simulink model "dcMotorControlSimPIDcode_2018b"  (R2018b)
settings: Solver=ode15s  StartTime=0.0  StopTime=10.0  RelTol=1e-3
PreLoadFcn:
  | dcMotorControlInit
undefined symbols (not defined in the file): sampleTime
libraries: fl_lib x16, nesl_utility x8, elec_lib x4, simulink x1, sdl_lib x1
Description:
  | DC Motor Control Simulation
settings Model: Creator=ControlLab  LastModifiedBy=arkadira
settings DataIOCC: SaveFormat=Array  SaveOutput=off  SignalLogging=off  DSMLogging=off  SaveTime=off

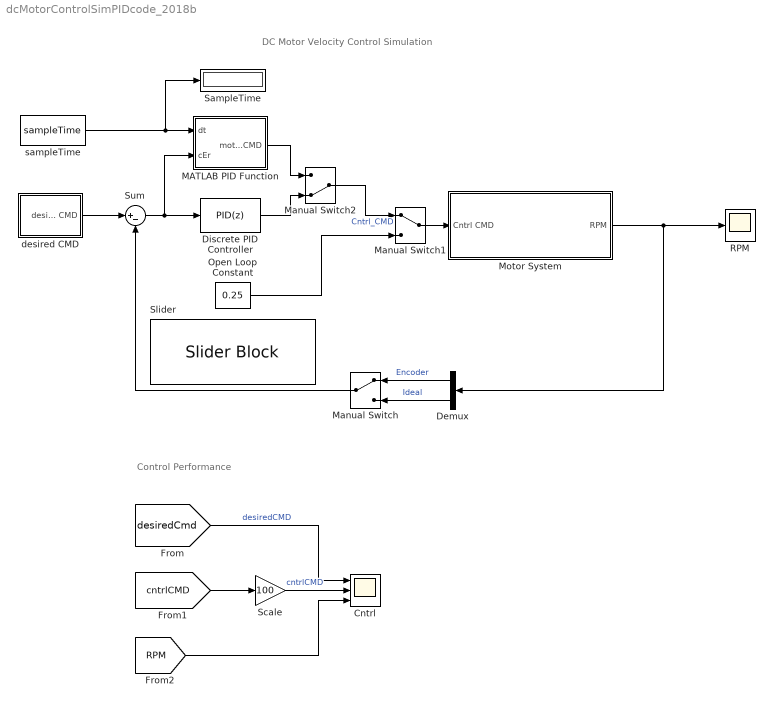
== system dcMotorControlSimPIDcode_2018b ==
  note: Control Performance
  note: DC Motor Velocity Control Simulation
  Cntrl : Scope  NumInputPorts=3
  Demux : Demux  Outputs=2
  Discrete PID Controller : simulink/Continuous/PID Controller  Controller=PID  Form=Parallel  TimeDomain=Discrete-time  SampleTime=sampleTime  IntegratorMethod=Forward Euler  FilterMethod=Forward Euler  ControllerParametersSource=internal  P=0.025  I=0.05  D=0.0001  UseFilter=off  N=0  TunerSelectOption=Transfer Function Based (PID Tuner App)  InitialConditionSource=internal  InitialConditionForIntegrator=0  InitialConditionForFilter=0  DifferentiatorICPrevScaledInput=0  ExternalReset=none  TrackingMode=off  Kt=1  LimitOutput=on  UpperSaturationLimit=1  LowerSaturationLimit=-1  LinearizeAsGain=on  AntiWindupMode=back-calculation  Kb=1  POutMin=[]  POutMax=[]  IOutMin=[]  IOutMax=[]  DOutMin=[]  DOutMax=[]  NOutMin=[]  NOutMax=[]  SumOutMin=[]  SumOutMax=[]  SaturationOutMin=[]  SaturationOutMax=[]  PParamMin=[]  PParamMax=[]  IParamMin=[]  IParamMax=[]  DParamMin=[]  DParamMax=[]  NParamMin=[]  NParamMax=[]  KbParamMin=[]  KbParamMax=[]  KtParamMin=[]  KtParamMax=[]  KbOutMin=[]  KbOutMax=[]  KtOutMin=[]  KtOutMax=[]  IntegratorOutMin=[]  IntegratorOutMax=[]  FilterOutMin=[]  FilterOutMax=[]  SumI1OutMin=[]  SumI1OutMax=[]  SumI2OutMin=[]  SumI2OutMax=[]  SumI3OutMin=[]  SumI3OutMax=[]  SumI4OutMin=[]  SumI4OutMax=[]  SumDOutMin=[]  SumDOutMax=[]  DifferentiatorOutMin=[]  DifferentiatorOutMax=[]  FilterDiffOutCoefMin=[]  FilterDiffOutCoefMax=[]  ReciprocalOutMin=[]  ReciprocalOutMax=[]  SumDenOutMin=[]  SumDenOutMax=[]  SumNumOutMin=[]  SumNumOutMax=[]  DivideOutMin=[]  DivideOutMax=[]  IntegratorContinuousStateAttributes=''  IntegratorStateMustResolveToSignalObject=off  IntegratorRTWStateStorageClass=Auto  FilterContinuousStateAttributes=''  FilterStateMustResolveToSignalObject=off  FilterRTWStateStorageClass=Auto  ParallelPVariant=InternalParameters  IdealPVariant=Disabled  IVariant=InternalParameters  DVariant=InternalParameters  IntegratorVariant=Discrete  SatVariant=Enabled  AWVariant=BackCalculation  PCopyVariant=Disabled  TRVariant=Disabled  FdbkBlocksVariant=Forward  IdealPFdbkVariant=Disabled  SatFdbkVariant=Disabled  DerivativeFilterVariant=Differentiator  NVariant=Passthrough  NCopyVariant=Disabled_SignalSpec  FilterICVariant=InternalICsDifferentiator  IntegratorICVariant=InternalICs  ExternalResetVariant=Disabled  TRSumVariant=Passthrough  SumFdbkVariant=Disabled  SumVariant=Sum_PID
  MATLAB PID Function : MATLAB Function  TreatAsAtomicUnit=on  SystemSampleTime=sampleTime
  Manual Switch : ManualSwitch
  Manual Switch1 : ManualSwitch
  Manual Switch2 : ManualSwitch  CurrentSetting=0
  Motor System : Subsystem
  Open Loop Constant : Constant  Value=0.25  SampleTime=sampleTime
  RPM : Scope
  SampleTime : Display
  Scale : Gain  Gain=100
  Slider : SliderBlock  WebBlockId=102  ScaleMin=-1  ScaleMax=1
  Sum : Sum  Inputs=|+-
  desired CMD : Subsystem
  sampleTime : Constant  Value=sampleTime  SampleTime=sampleTime
  wires:
  Open Loop Constant/1 -> Manual Switch1/2
  Manual Switch1/1 -> Motor System/1(Cntrl CMD)
  Sum/1 -> MATLAB PID Function/2(cEr), Discrete PID Controller/1
  Demux/2 -> Manual Switch/2  "Ideal"
  desired CMD/1(desired CMD) -> Sum/1
  Motor System/1(RPM) -> Demux/1, RPM/1
  Manual Switch/1 -> Sum/2
  Demux/1 -> Manual Switch/1  "Encoder"
  sampleTime/1 -> SampleTime/1, MATLAB PID Function/1(dt)
  [desiredCmd] -> Cntrl/1  "desiredCMD"
  [cntrlCMD] -> Scale/1
  Scale/1 -> Cntrl/2  "cntrlCMD"
  [RPM] -> Cntrl/3
  Manual Switch2/1 -> Manual Switch1/1  "Cntrl_CMD"
  Discrete PID Controller/1 -> Manual Switch2/2
  MATLAB PID Function/1(motorCMD) -> Manual Switch2/1

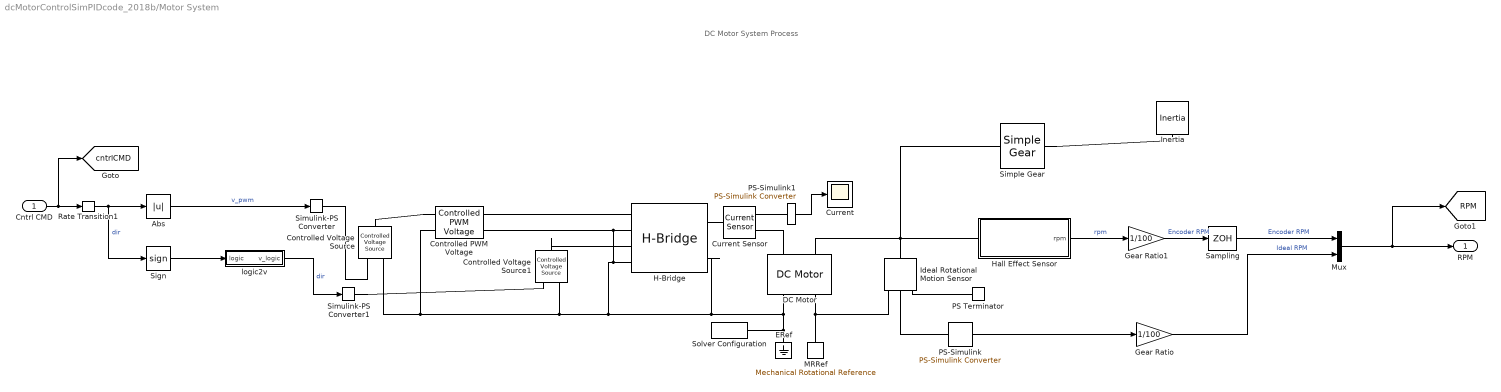
== system dcMotorControlSimPIDcode_2018b/Motor System ==
  note: DC Motor System Process
  Cntrl CMD : Inport
  Abs : Abs
  Controlled PWM Voltage : elec_lib/Actuators & Drivers/Drivers/Controlled PWM Voltage  F=512 Hz  TD=0 s  pulse_width_offset=0 s  pulse_min=0 s  Vmin=0 V  Vmax=1 V  Vm=5 V  pwm_or_av=2  event_type=1  sample_time=1e-6 s  u_min=0  u_max=1
      settings: SourceProductName=Simscape Electronics  SourceProductBaseCode=SN
  Controlled Voltage Source : fl_lib/Electrical/Electrical Sources/Controlled Voltage Source
  Controlled Voltage Source1 : fl_lib/Electrical/Electrical Sources/Controlled Voltage Source
  Current : Scope
  Current Sensor : fl_lib/Electrical/Electrical Sensors/Current Sensor
      settings: SourceProductBaseCode=MT,SS
  DC Motor : elec_lib/Actuators & Drivers/Rotational Actuators/DC Motor  parameterization=2  Ra=3.9 Ohm  La=0.5 mH  emf_or_torque=1  Kv=0.072e-3 V/rpm  Ki=6.876e-4 N*m/A  T_stall=0.001274 N*m  w_max=33000 rpm  w_rated=15000 rpm  P_rated=0.08 W  V_rated=12 V  J=1 g*cm^2  lam_param=2  lam=0 N*m/(rad/s)  i_noload=0.054 A  V_i_noload=2.5 V  speed0=0 rpm  alpha=3.93e-3 1/K  Tmeas=25 degC  thermal_mass=100 J/K  initial_temperature=25 degC
  ERef : fl_lib/Electrical/Electrical Elements/Electrical Reference
      settings: SourceProductBaseCode=MT,SS
  Gear Ratio : Gain  Gain=1/100
  Gear Ratio1 : Gain  Gain=1/100
  H-Bridge : elec_lib/Actuators & Drivers/Drivers/H-Bridge  Venable=2.5 V  Vmax=5.0 V  Vreverse=2.5 V  Vbrake=2.5 V  Vm=12 V  pwm_or_av=2  discontinuous=0  freewheeling_mode=1  freewheeling_mode_disc=1  Ron=0.1 Ohm  Don=0.1 Ohm  Rload=10 Ohm  Lload=1e-5 H  F=10 kHz  thermal_mass=100 J/K  initial_temperature=298.15 K  Ron2=0.1 Ohm  Don2=0.05 Ohm  Tmeas=298.15 K  Tmeas2=398.15 K
      settings: SourceProductName=Simscape Electronics  SourceProductBaseCode=SN
  Hall Effect Sensor : Subsystem
  Ideal Rotational Motion Sensor : fl_lib/Mechanical/Mechanical Sensors/Ideal Rotational Motion Sensor  offset=0 deg
      settings: SourceProductBaseCode=MT,SS
  Inertia : fl_lib/Mechanical/Rotational Elements/Inertia  inertia=50 g*cm^2  w_specify=on  w_priority=None  w=0 rad/s  w_nominal_specify=off  w_nominal_unit=rad/s  w_nominal_value=1  t_specify=off  t_priority=High  t=0 N*m  t_nominal_specify=off  t_nominal_unit=N*m  t_nominal_value=1
      settings: SourceProductBaseCode=MT,SS
  MRRef : fl_lib/Mechanical/Rotational Elements/Mechanical Rotational Reference
      settings: SourceProductBaseCode=MT,SS
  Mux : Mux  Inputs=2
  PS Terminator : fl_lib/Physical Signals/Sinks/PS Terminator
      settings: SourceProductName=Simscape
  PS-Simulink : nesl_utility/PS-Simulink Converter  PhysicalDomain=network_engine_domain  SubClassName=ps_output  LeftPortType=input  RightPortType=output  PseudoPeriodic=off  Frequencies=[]  Unit=rpm  AffineConversion=off
      settings: SourceProductBaseCode=MT,SS
  PS-Simulink1 : nesl_utility/PS-Simulink Converter  PhysicalDomain=network_engine_domain  SubClassName=ps_output  LeftPortType=input  RightPortType=output  PseudoPeriodic=off  Frequencies=[]  Unit=A  AffineConversion=off
      settings: SourceProductBaseCode=MT,SS
  Rate Transition1 : RateTransition
  Sampling : ZeroOrderHold  SampleTime=sampleTime
  Sign : Signum
  Simple Gear : sdl_lib/Gears/Simple Gear  ratio=100  rotation_direction=1  friction_model=sdl.enum.gear_efficiencies_load.constant  T_noload=0.1 N*m  T_nom=5 N*m  efficiency_nom=0.8  efficiency=0.24  mu_visc=[0, 0] N*m/(rad/s)  w_thr=0.01 rad/s  pwr_thr=0.1 W  enable_faults=simscape.enum.onoff.off  efficiency_fault=0.05  external_fault=simscape.enum.onoff.off  temporal_fault=simscape.enum.onoff.off  fault_time=5 s  fault_angles=pi / 12 rad  report_fault=1  temperature_TLU=[280, 300, 320] K  load_TLU=[1, 5, 10] N*m  efficiency_TLU=[.95, .9, .85]  efficiency_TLU2=[.85, .8, .75; .95, .9, .85; .85, .8, .7]  thermal_mass=50 J/K  T_init=300 K
  Simulink-PS Converter : nesl_utility/Simulink-PS Converter  PhysicalDomain=network_engine_domain  SubClassName=ps_input  LeftPortType=input  RightPortType=output  PseudoPeriodic=off  Frequencies=[]  NoiseDistribution=none  NoiseParameters=[]  Unit=1  AffineConversion=off  FilteringAndDerivatives=provide  SimscapeFilterOrder=1  InputFilterTimeConstant=0.001  UdotUserProvided=0
  Simulink-PS Converter1 : nesl_utility/Simulink-PS Converter  PhysicalDomain=network_engine_domain  SubClassName=ps_input  LeftPortType=input  RightPortType=output  PseudoPeriodic=off  Frequencies=[]  NoiseDistribution=none  NoiseParameters=[]  Unit=1  AffineConversion=off  FilteringAndDerivatives=provide  SimscapeFilterOrder=1  InputFilterTimeConstant=0.001  UdotUserProvided=0
  Solver Configuration : nesl_utility/Solver Configuration  PhysicalDomain=network_engine_domain  SubClassName=solver  LeftPortType=input  RightPortType=generic  Tones=[]  Harmonics=[]  SimulateNoise=off  Profile=off  UseLocalSampling=off  EnableSwitchedLinearOptims=on  FrequencyDomain=off  UseCCode=off  RelTol=0.001  AbsTol=1e-06  MinStep=1e-09  ToWorkspace=off  RevertToSquareIcSolve=off  NumHomotopyIterations=100  PhasorMode=off  PhasorModeNumHarmonics=1  DoDC=off  ResidualTolerance=1e-9  UseLocalSolver=off  LocalSolverChoice=NE_BACKWARD_EULER_ADVANCER  LocalSolverSampleTime=5e-6  DoFixedCost=off  MaxNonlinIter=4  MaxModeIter=2  LinearAlgebra=auto  EquationFormulation=NE_TIME_EF  DelaysMemoryBudget=1024  AutomaticFiltering=on  FilteringTimeConstant=0.001  PartitionStorageMethod=AS_NEEDED  PartitionMemoryBudget=1024
      settings: SourceProductBaseCode=MT,SS
  logic2v : Subsystem
  RPM : Outport  VectorParamsAs1DForOutWhenUnconnected=on
  tag scope: RPM=global, cntrlCMD=global
  wires:
  logic2v/1(v_logic) -> Simulink-PS Converter1/1  "dir"
  PS-Simulink1/1 -> Current/1
  Hall Effect Sensor/1(rpm) -> Gear Ratio1/1  "rpm"
  Gear Ratio1/1 -> Sampling/1  "Encoder RPM"
  Gear Ratio/1 -> Mux/2  "Ideal RPM"
  PS-Simulink/1 -> Gear Ratio/1
  Mux/1 -> [RPM], RPM/1
  Cntrl CMD/1 -> [cntrlCMD], Rate Transition1/1
  Abs/1 -> Simulink-PS Converter/1  "v_pwm"
  Sign/1 -> logic2v/1(logic)
  Rate Transition1/1 -> Sign/1, Abs/1  "dir"
  Sampling/1 -> Mux/1  "Encoder RPM"
  connections:
  PS Terminator/LConn1 -- Ideal Rotational Motion Sensor/RConn3
  Controlled PWM Voltage/LConn1 -- Controlled Voltage Source/LConn1
  Controlled Voltage Source/RConn2 -- Controlled PWM Voltage/LConn2 -- Controlled Voltage Source1/RConn2 -- H-Bridge/RConn2 -- DC Motor/RConn1 -- Solver Configuration/RConn1 -- ERef/LConn1 -- H-Bridge/LConn4 -- Controlled PWM Voltage/RConn2 -- H-Bridge/LConn2
  MRRef/LConn1 -- DC Motor/RConn2 -- Ideal Rotational Motion Sensor/RConn1
  H-Bridge/RConn1 -- Current Sensor/LConn1
  DC Motor/LConn1 -- Current Sensor/RConn2
  Simple Gear/LConn1 -- DC Motor/LConn2 -- Ideal Rotational Motion Sensor/LConn1 -- Hall Effect Sensor/LConn1
  Controlled Voltage Source1/LConn1 -- H-Bridge/LConn3
  Simulink-PS Converter/RConn1 -- Controlled Voltage Source/RConn1
  Current Sensor/RConn1 -- PS-Simulink1/LConn1
  Simulink-PS Converter1/RConn1 -- Controlled Voltage Source1/RConn1
  PS-Simulink/LConn1 -- Ideal Rotational Motion Sensor/RConn2
  Simple Gear/RConn1 -- Inertia/LConn1
  Controlled PWM Voltage/RConn1 -- H-Bridge/LConn1

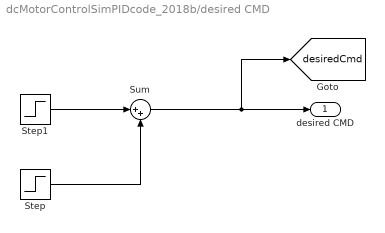
== system dcMotorControlSimPIDcode_2018b/desired CMD ==
  Step : Step  Time=7  After=-100  SampleTime=sampleTime
  Step1 : Step  After=100  SampleTime=sampleTime
  Sum : Sum  Inputs=|++
  desired CMD : Outport  VectorParamsAs1DForOutWhenUnconnected=on
  tag scope: desiredCmd=global
  wires:
  Step/1 -> Sum/2
  Step1/1 -> Sum/1
  Sum/1 -> [desiredCmd], desired CMD/1

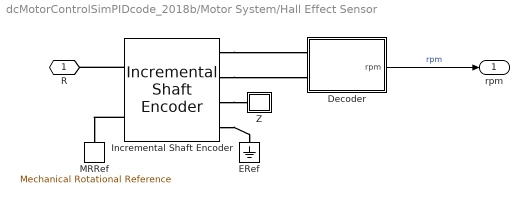
== system dcMotorControlSimPIDcode_2018b/Motor System/Hall Effect Sensor ==
  Decoder : Subsystem
  ERef : fl_lib/Electrical/Electrical Elements/Electrical Reference
      settings: SourceProductBaseCode=MT,SS
  Incremental Shaft Encoder : elec_lib/Sensors/Incremental Shaft Encoder  NPulse=3  Vm=5 V  angle0=-1 deg
      settings: SourceProductName=Simscape Electronics  SourceProductBaseCode=SN
  MRRef : fl_lib/Mechanical/Rotational Elements/Mechanical Rotational Reference
      settings: SourceProductBaseCode=MT,SS
  Z : Subsystem
  R : PMIOPort  Side=Left
  rpm : Outport
  wires:
  Decoder/1(rpm) -> rpm/1  "rpm"
  connections:
  Incremental Shaft Encoder/LConn2 -- MRRef/LConn1
  Incremental Shaft Encoder/LConn1 -- R/RConn1
  Incremental Shaft Encoder/RConn4 -- ERef/LConn1
  Incremental Shaft Encoder/RConn3 -- Z/LConn1
  Incremental Shaft Encoder/RConn2 -- Decoder/LConn2
  Incremental Shaft Encoder/RConn1 -- Decoder/LConn1

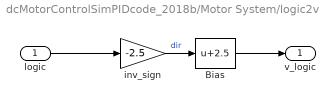
== system dcMotorControlSimPIDcode_2018b/Motor System/logic2v ==
  logic : Inport
  Bias : Bias  Bias=2.5
  inv_sign : Gain  Gain=-2.5
  v_logic : Outport  VectorParamsAs1DForOutWhenUnconnected=on
  wires:
  inv_sign/1 -> Bias/1  "dir"
  logic/1 -> inv_sign/1
  Bias/1 -> v_logic/1

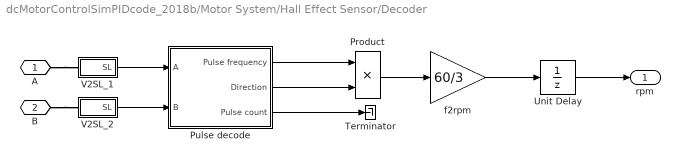
== system dcMotorControlSimPIDcode_2018b/Motor System/Hall Effect Sensor/Decoder ==
  Product : Product  RndMeth=Zero
  Pulse decode : Subsystem
  Terminator : Terminator
  Unit Delay : UnitDelay  SampleTime=sampleTime
  V2SL_1 : Subsystem
  V2SL_2 : Subsystem
  f2rpm : Gain  Gain=60/3
  A : PMIOPort  Side=Left
  B : PMIOPort  Port=2  Side=Left
  rpm : Outport
  wires:
  Product/1 -> f2rpm/1
  Pulse decode/2(Direction) -> Product/2
  Pulse decode/1(Pulse frequency) -> Product/1
  Pulse decode/3(Pulse count) -> Terminator/1
  V2SL_1/1(SL) -> Pulse decode/1(A)
  V2SL_2/1(SL) -> Pulse decode/2(B)
  f2rpm/1 -> Unit Delay/1
  Unit Delay/1 -> rpm/1
  connections:
  A/RConn1 -- V2SL_1/LConn1
  B/RConn1 -- V2SL_2/LConn1

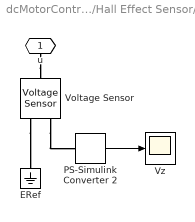
== system dcMotorControlSimPIDcode_2018b/Motor System/Hall Effect Sensor/Z ==
  ERef : fl_lib/Electrical/Electrical Elements/Electrical Reference
      settings: SourceProductBaseCode=MT,SS
  PS-Simulink Converter 2 : nesl_utility/PS-Simulink Converter  PhysicalDomain=network_engine_domain  SubClassName=ps_output  LeftPortType=input  RightPortType=output  PseudoPeriodic=off  Frequencies=[]  Unit=V  AffineConversion=off
      settings: SourceProductBaseCode=MT,SS
  Voltage Sensor : fl_lib/Electrical/Electrical Sensors/Voltage Sensor
      settings: SourceProductBaseCode=MT,SS
  Vz : Scope
  u : PMIOPort  Side=Left
  wires:
  PS-Simulink Converter 2/1 -> Vz/1
  connections:
  Voltage Sensor/RConn2 -- ERef/LConn1
  Voltage Sensor/RConn1 -- PS-Simulink Converter 2/LConn1
  u/RConn1 -- Voltage Sensor/LConn1

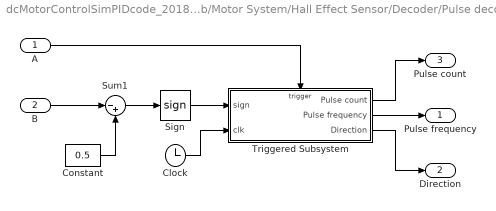
== system dcMotorControlSimPIDcode_2018b/Motor System/Hall Effect Sensor/Decoder/Pulse decode ==
  A : Inport
  B : Inport  Port=2
  Clock : Clock
  Constant : Constant  Value=0.5
  Sign : Signum
  Sum1 : Sum  Inputs=|-+
  Triggered Subsystem : Subsystem  TreatAsAtomicUnit=on
  Pulse frequency : Outport
  Direction : Outport  Port=2
  Pulse count : Outport  Port=3
  wires:
  Triggered Subsystem/3(Direction) -> Direction/1
  Triggered Subsystem/2(Pulse frequency) -> Pulse frequency/1
  Clock/1 -> Triggered Subsystem/2(clk)
  Triggered Subsystem/1(Pulse count) -> Pulse count/1
  A/1 -> Triggered Subsystem/Trigger
  Sign/1 -> Triggered Subsystem/1(sign)
  B/1 -> Sum1/1
  Sum1/1 -> Sign/1
  Constant/1 -> Sum1/2

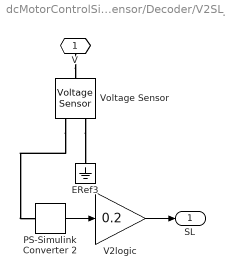
== system dcMotorControlSimPIDcode_2018b/Motor System/Hall Effect Sensor/Decoder/V2SL_1 ==
  ERef3 : fl_lib/Electrical/Electrical Elements/Electrical Reference
      settings: SourceProductBaseCode=MT,SS
  PS-Simulink Converter 2 : nesl_utility/PS-Simulink Converter  PhysicalDomain=network_engine_domain  SubClassName=ps_output  LeftPortType=input  RightPortType=output  PseudoPeriodic=off  Frequencies=[]  Unit=V  AffineConversion=off
      settings: SourceProductBaseCode=MT,SS
  V2logic : Gain  Gain=0.2
  Voltage Sensor : fl_lib/Electrical/Electrical Sensors/Voltage Sensor
      settings: SourceProductBaseCode=MT,SS
  V : PMIOPort  Side=Left
  SL : Outport
  wires:
  PS-Simulink Converter 2/1 -> V2logic/1
  V2logic/1 -> SL/1
  connections:
  Voltage Sensor/RConn2 -- ERef3/LConn1
  V/RConn1 -- Voltage Sensor/LConn1
  Voltage Sensor/RConn1 -- PS-Simulink Converter 2/LConn1

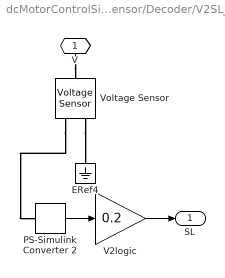
== system dcMotorControlSimPIDcode_2018b/Motor System/Hall Effect Sensor/Decoder/V2SL_2 ==
  ERef4 : fl_lib/Electrical/Electrical Elements/Electrical Reference
      settings: SourceProductBaseCode=MT,SS
  PS-Simulink Converter 2 : nesl_utility/PS-Simulink Converter  PhysicalDomain=network_engine_domain  SubClassName=ps_output  LeftPortType=input  RightPortType=output  PseudoPeriodic=off  Frequencies=[]  Unit=V  AffineConversion=off
      settings: SourceProductBaseCode=MT,SS
  V2logic : Gain  Gain=0.2
  Voltage Sensor : fl_lib/Electrical/Electrical Sensors/Voltage Sensor
      settings: SourceProductBaseCode=MT,SS
  V : PMIOPort  Side=Left
  SL : Outport
  wires:
  V2logic/1 -> SL/1
  PS-Simulink Converter 2/1 -> V2logic/1
  connections:
  Voltage Sensor/RConn1 -- PS-Simulink Converter 2/LConn1
  V/RConn1 -- Voltage Sensor/LConn1
  Voltage Sensor/RConn2 -- ERef4/LConn1

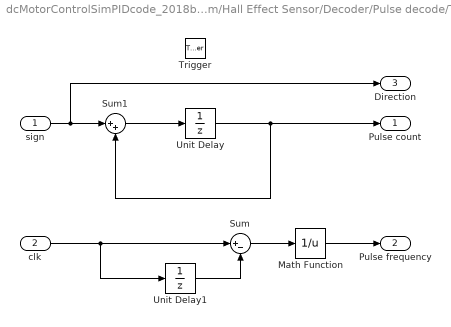
== system dcMotorControlSimPIDcode_2018b/Motor System/Hall Effect Sensor/Decoder/Pulse decode/Triggered Subsystem ==
  sign : Inport
  clk : Inport  Port=2
  Trigger : TriggerPort  VariantControl=Variant
  Math Function : Math  Operator=reciprocal  SaturateOnIntegerOverflow=on
  Sum : Sum  Inputs=|+-
  Sum1 : Sum  Inputs=|++
  Unit Delay : UnitDelay  SampleTime=-1
  Unit Delay1 : UnitDelay  InitialCondition=-1e10  SampleTime=-1
  Pulse count : Outport  InitialOutput=0
  Pulse frequency : Outport  Port=2
  Direction : Outport  Port=3  InitialOutput=0
  wires:
  Math Function/1 -> Pulse frequency/1
  Sum/1 -> Math Function/1
  Unit Delay1/1 -> Sum/2
  clk/1 -> Sum/1, Unit Delay1/1
  Unit Delay/1 -> Sum1/2, Pulse count/1
  sign/1 -> Direction/1, Sum1/1
  Sum1/1 -> Unit Delay/1

== matlab function dcMotorControlSimPIDcode_2018b/MATLAB PID Function ==
  data: dt input; cEr input; motorCMD output
function motorCMD = PID(dt,cEr)
% persistant variables persist between function calls. similar to static
% variable declaration in c
persistent lEr cdEr ciEr; 
if isempty(lEr) %initialize variables for first run of the code.
  lEr = 0;  % previous error initialization
  cdEr = 0; % differantional error initialization
  ciEr = 0; % integral error initialization
end
% control coeficients
kp = 0.025;




% clip integrator error
   if (ciEr > 10) 
       ciEr = 10;
   elseif (ciEr < -10) 
       ciEr = -10;
   end 

% update control command
motorCMD = kp*cEr;
  
% clip motor command
   if (motorCMD > 1) 
       motorCMD = 1;
   elseif (motorCMD < -1) 
       motorCMD = -1;
   end
   
% update last error variable before next iteration
lEr = cEr;
